simulink model "vehicle_simulationV2"  (R2020a)
settings: Solver=ode1  StartTime=0.0  StopTime=500  FixedStep=0.1  RelTol=1e-3
undefined symbols (not defined in the file): HDBK, MIL, serial
libraries: powerlib_meascontrol x7, aerolibconvert2 x5, aerolibatmos2 x3, instrumentlib x3, dspsrcs4 x2, simulink x1
(part 1 of 6)
settings Model: SimulationMode=accelerator  EnablePacing=on  Creator=Jared  LastModifiedBy=Mason
settings SolverCC: DecoupledContinuousIntegration=on  MinimalZcImpactIntegration=on
settings DataIOCC: SaveOutput=off  SignalLogging=off  DSMLogging=off  SaveTime=off  ReturnWorkspaceOutputs=off
settings DebuggingCC: ArithmeticOperatorsInVariantConditions=warning
settings SFSimCC: SimUseLocalCustomCode=off  CustomCodeUndefinedFunction=UseInterfaceOnly
settings RTWCC: RTWUseLocalCustomCode=off

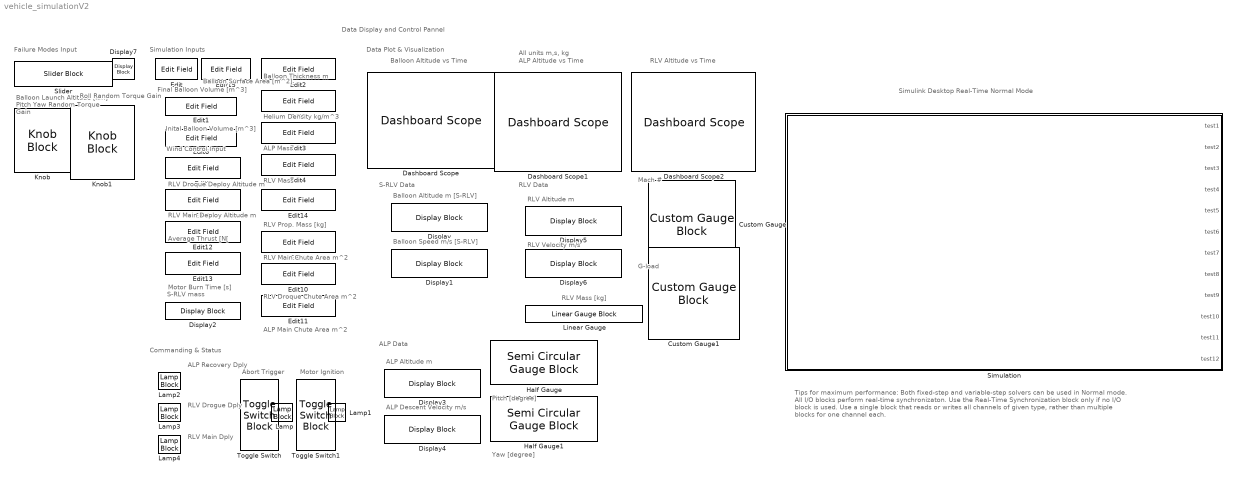
== system vehicle_simulationV2 ==
  note: Failure Modes Input
  note: RLV Mass [kg]
  note: RLV Data
  note: Mach #
  note: ALP Data
  note: S-RLV Data
  note: Data Plot & Visualization
  note: Commanding & Status
  note: Simulation Inputs
  note: Tips for maximum performance:
      |
      | Both fixed-step and variable-step solvers can be used in Normal mode.
      | All I/O blocks perform real-time synchronizaton. Use the Real-Time Synchronization block only if no I/O block is used.
      | Use a single block that reads or writes all channels of given type, rather than multiple blocks for one channel each.
  note: Data Display and Control Pannel
  note: Simulink Desktop Real-Time Normal Mode
  note: Inital Balloon Volume [m^3]
  note: Final Balloon Volume [m^3]
  note: Abort Trigger
  note: Motor Ignition
  note: Balloon Thickness m
  note: ALP Mass
  note: RLV Mass
  note: Helium Density kg/m^3
  note: Balloon Altitude vs Time
  note: Balloon Altitude m [S-RLV]
  note: Balloon Speed m/s [S-RLV]
  note: Wind Control Input
  note: S-RLV mass
  note: ALP Altitude m
  note: ALP Descent Velocity m/s
  note: ALP Recovery Dply
  note: RLV Droque Deploy Altitude m
  note: RLV Main Deploy Altitude m
  note: RLV Main Chute Area m^2
  note: RLV Droque Chute Area m^2
  note: ALP Main Chute Area m^2
  note: RLV Drogue Dply
  note: RLV
      | Main
      | Dply
  note: RLV Velocity m/s
  note: RLV Altitude m
  note: Average Thrust [N[
  note: Motor Burn Time [s]
  note: RLV Prop. Mass [kg]
  note: ALP Altitude vs Time
  note: RLV Altitude vs Time
  note: All units m,s, kg
  note: Balloon Surface Area [m^2]
  note: Balloon Launch Altitude [km]
  note: G-load
  note: Pitch Yaw Random Torque Gain
  note: Roll Random Torque Gain
  note: Pitch [degree]
  note: Yaw [degree]
  Custom Gauge : CustomGaugeBlock  LabelPosition=Hide  NeedleImage=data:image/svg+xml;base64,PD94bWwgdmVyc2lvbj0iMS4wIiBlbmNvZGluZz0idXRmLTgiPz4KPCEtLSBHZW5lcmF0b3I6IEFkb2JlIElsbHVzdHJhdG9yIDE5LjIuMSwgU1ZHIEV4cG9ydCBQbHVnLUluIC4gU1ZHIFZlcnNpb246IDYuMDAgQnVpbGQgMCkgIC0tPgo8c3ZnIHZlcnNpb249IjEuMSIgeG1sbnM9Imh0dHA6Ly93d3cudzMub3JnLzIwMDAvc3ZnIiB4bWxuczp4bGluaz0iaHR0cDovL3d3dy53My5vcmcvMTk5OS94bGluayIgeD0iMHB4IiB5PSIwcHgiCgkgdmlld0JveD0iMCAwIDIwMCA1MCIgc3R5bGU9ImVuYWJsZS1iYWNrZ3JvdW5kOm5ldyAw ...(+9940 chars)  NeedleXPos=0.3802298124325669  NeedleYPos=0.483542725020692  NeedleHeight=0.11602152693163792  NeedleWidth=0.1911368983686954  NeedleInitialRotation=-59.94322499147643  BackgroundImage=data:image/svg+xml;base64,PD94bWwgdmVyc2lvbj0iMS4wIiBlbmNvZGluZz0iVVRGLTgiIHN0YW5kYWxvbmU9Im5vIj8+CjwhLS0gR2VuZXJhdG9yOiBBZG9iZSBJbGx1c3RyYXRvciAxOS4yLjEsIFNWRyBFeHBvcnQgUGx1Zy1JbiAuIFNWRyBWZXJzaW9uOiA2LjAwIEJ1aWxkIDApICAtLT4KCjxzdmcKICAgeG1sbnM6ZGM9Imh0dHA6Ly9wdXJsLm9yZy9kYy9lbGVtZW50cy8xLjEvIgogICB4bWxuczpjYz0iaHR0cDovL2NyZWF0aXZlY29tbW9ucy5vcmcvbnMjIgogICB4bWxuczpyZGY9Imh0dHA6Ly93d3cudzMub3JnLzE5OTkvMDIvMjItcmRmLXN5bnRh ...(+9660 chars)  GaugeMax=5  GaugeArcDefined=true  GaugeArcRadius=0.1411189948569805  GaugeArcStrokeWidth=0.029204463724193906  GaugeArcRotation=240.5385250290321  GaugeArcRatio=0.8333333333333  GaugeArcTransparency=0  ValueArcColor=#1759b0  GaugeTickColor=#faf5c8  ScaleColorsJSON=[]  fixedAspectRatio=on
  Custom Gauge1 : CustomGaugeBlock  LabelPosition=Hide  NeedleImage=data:image/svg+xml;base64,PD94bWwgdmVyc2lvbj0iMS4wIiBlbmNvZGluZz0idXRmLTgiPz4KPCEtLSBHZW5lcmF0b3I6IEFkb2JlIElsbHVzdHJhdG9yIDE5LjIuMSwgU1ZHIEV4cG9ydCBQbHVnLUluIC4gU1ZHIFZlcnNpb246IDYuMDAgQnVpbGQgMCkgIC0tPgo8c3ZnIHZlcnNpb249IjEuMSIgeG1sbnM9Imh0dHA6Ly93d3cudzMub3JnLzIwMDAvc3ZnIiB4bWxuczp4bGluaz0iaHR0cDovL3d3dy53My5vcmcvMTk5OS94bGluayIgeD0iMHB4IiB5PSIwcHgiCgkgdmlld0JveD0iMCAwIDIwMCA1MCIgc3R5bGU9ImVuYWJsZS1iYWNrZ3JvdW5kOm5ldyAw ...(+9940 chars)  NeedleXPos=0.3802298124325669  NeedleYPos=0.483542725020692  NeedleHeight=0.11602152693163792  NeedleWidth=0.1911368983686954  NeedleInitialRotation=-59.94322499147643  BackgroundImage=data:image/svg+xml;base64,PD94bWwgdmVyc2lvbj0iMS4wIiBlbmNvZGluZz0iVVRGLTgiIHN0YW5kYWxvbmU9Im5vIj8+CjwhLS0gR2VuZXJhdG9yOiBBZG9iZSBJbGx1c3RyYXRvciAxOS4yLjEsIFNWRyBFeHBvcnQgUGx1Zy1JbiAuIFNWRyBWZXJzaW9uOiA2LjAwIEJ1aWxkIDApICAtLT4KCjxzdmcKICAgeG1sbnM6ZGM9Imh0dHA6Ly9wdXJsLm9yZy9kYy9lbGVtZW50cy8xLjEvIgogICB4bWxuczpjYz0iaHR0cDovL2NyZWF0aXZlY29tbW9ucy5vcmcvbnMjIgogICB4bWxuczpyZGY9Imh0dHA6Ly93d3cudzMub3JnLzE5OTkvMDIvMjItcmRmLXN5bnRh ...(+9660 chars)  GaugeMax=40  GaugeArcDefined=true  GaugeArcRadius=0.1411189948569805  GaugeArcStrokeWidth=0.029204463724193906  GaugeArcRotation=240.5385250290321  GaugeArcRatio=0.8333333333333  GaugeArcTransparency=0  ValueArcColor=#1759b0  GaugeTickColor=#faf5c8  ScaleColorsJSON=[]  fixedAspectRatio=on
  Dashboard Scope : DashboardScope  Ymin=0  Ymax=28000  LegendPosition=Hide
  Dashboard Scope1 : DashboardScope  Ymin=0  Ymax=28000  LegendPosition=Hide
  Dashboard Scope2 : DashboardScope  Ymin=0  Ymax=110000  LegendPosition=Hide
  Display{,1..7} (8 alike) : DisplayBlock  LabelPosition=Hide
  Edit{,1..15} (16 alike) : EditField  LabelPosition=Hide  ShowInitialText=on  Alignment=Center
  Half Gauge : SemiCircularGaugeBlock  LabelPosition=Hide  ScaleMin=-10  ScaleMax=10
  Half Gauge1 : SemiCircularGaugeBlock  LabelPosition=Hide  ScaleMin=-10  ScaleMax=10
  Knob : KnobBlock  LabelPosition=Hide  ScaleMax=0.5
  Knob1 : KnobBlock  LabelPosition=Hide  ScaleMax=0.01
  Lamp{,1..4} (5 alike) : LampBlock  LabelPosition=Hide
  Linear Gauge : LinearGaugeBlock  LabelPosition=Hide  ScaleMin=20  ScaleMax=50
  Simulation : Subsystem  TreatAsAtomicUnit=on
  Slider : SliderBlock  LabelPosition=Hide  ScaleMax=25
  Toggle Switch : ToggleSwitchBlock  LabelPosition=Hide
      settings: Values={{'Off', 'On'}, [0 1]}
  Toggle Switch1 : ToggleSwitchBlock  LabelPosition=Hide
      settings: Values={{'Off', 'On'}, [0 1]}
